simulink model "launch_controller_base"  (R2024b)
settings: Solver=VariableStepAuto  StartTime=0.0  StopTime=10.0  FixedStep=0.004  RelTol=1e-3
settings Model: Creator=lukec  LastModifiedBy=lukec
settings OptimizationCC: DefaultParameterBehavior=Inlined  EnhancedBackFolding=on  PassReuseOutputArgsAs=Individual arguments  ZeroExternalMemoryAtStartup=off  ZeroInternalMemoryAtStartup=off  OptimizeBlockOrder=speed  DifferentSizesBufferReuse=on  OptimizationCustomize=off  EfficientTunableParamExpr=on
settings DebuggingCC: ParameterTunabilityLossMsg=error
settings SFSimCC: MATLABDynamicMemAlloc=off
settings RTWCC: Description=Embedded Coder  SystemTargetFile=ert.tlc  GenCodeOnly=on  PackageGeneratedCodeAndArtifacts=on  TemplateMakefile=ert_default_tmf  Toolchain=CMake  TargetLang=C++
settings CodeAppCC: ForceParamTrailComments=on  IgnoreCustomStorageClasses=off  OperatorAnnotations=on  SimulinkDataObjDesc=on  SFDataObjDesc=on  InsertBlockDesc=on
settings ERTTargetCC: TargetLangStandard=C++11 (ISO)  GenerateSampleERTMain=on  CodeInterfacePackaging=C++ class  RootIOFormat=Structure reference  ERTCustomFileTemplate=example_file_process.tlc

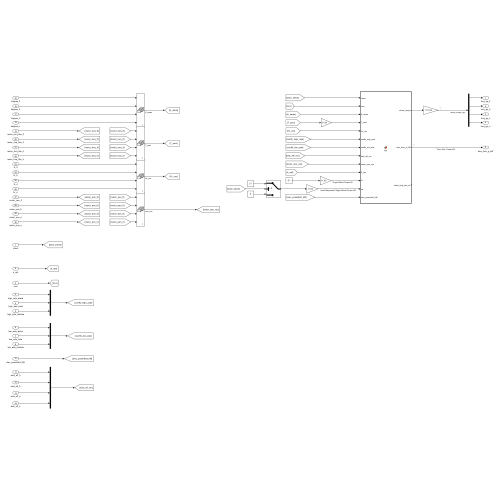
[thumbnail: Simulink's stored preview of the top-level diagram]
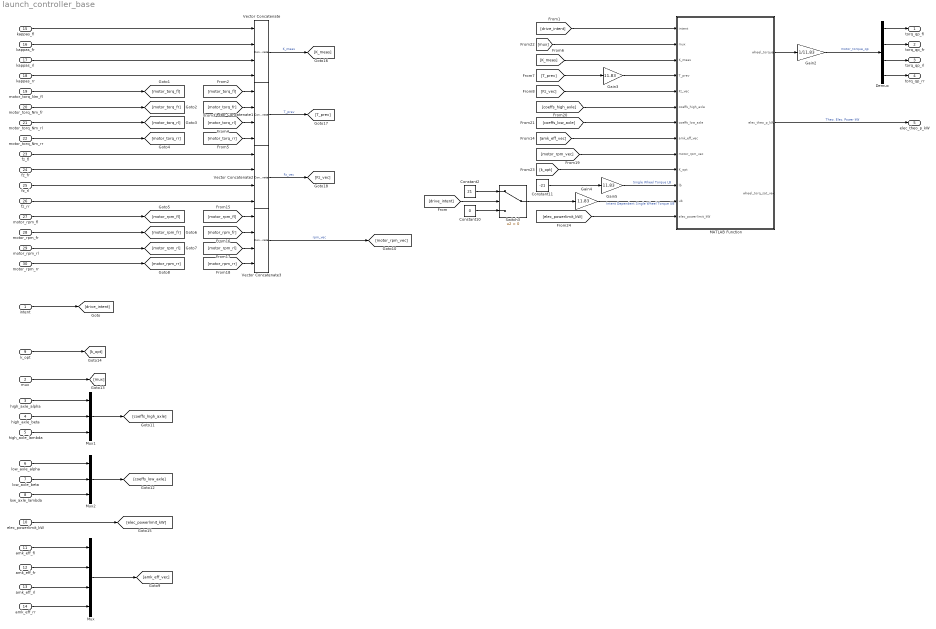
== system launch_controller_base ==
  intent : Inport
  mux : Inport  Port=2
  high_axle_alpha : Inport  Port=3
  high_axle_beta : Inport  Port=4
  high_axle_lambda : Inport  Port=5
  low_axle_alpha : Inport  Port=6
  low_axle_beta : Inport  Port=7
  low_axle_lambda : Inport  Port=8
  k_opt : Inport  Port=9
  elec_powerlimit_kW : Inport  Port=10
  amk_eff_fl : Inport  Port=11
  amk_eff_fr : Inport  Port=12
  amk_eff_rl : Inport  Port=13
  amk_eff_rr : Inport  Port=14
  kappas_fl : Inport  Port=15
  kappas_fr : Inport  Port=16
  kappas_rl : Inport  Port=17
  kappas_rr : Inport  Port=18
  motor_torq_Nm_fl : Inport  Port=19
  motor_torq_Nm_fr : Inport  Port=20
  motor_torq_Nm_rl : Inport  Port=21
  motor_torq_Nm_rr : Inport  Port=22
  fz_fl : Inport  Port=23
  fz_fr : Inport  Port=24
  fz_rl : Inport  Port=25
  fz_rr : Inport  Port=26
  motor_rpm_fl : Inport  Port=27
  motor_rpm_fr : Inport  Port=28
  motor_rpm_rl : Inport  Port=29
  motor_rpm_rr : Inport  Port=30
  Constant10 : Constant  Value=0
  Constant11 : Constant  Value=-21
  Constant2 : Constant  Value=21
  Demux : Demux
  Gain2 : Gain  Gain=1/11.83
  Gain3 : Gain  Gain=11.83
  Gain4 : Gain  Gain=11.83
  Gain5 : Gain  Gain=11.83
  MATLAB Function : MATLAB Function  TreatAsAtomicUnit=on
  Mux : Mux
  Mux1 : Mux  Inputs=3
  Mux2 : Mux  Inputs=3
  Switch3 : Switch  Criteria=u2 > Threshold  SaturateOnIntegerOverflow=off  InputSameDT=off
  Vector Concatenate{,1..3} (4 alike) : Concatenate  NumInputs=4  Mode=Multidimensional array
  torq_qp_fl : Outport
  torq_qp_fr : Outport  Port=2
  torq_qp_rl : Outport  Port=3
  torq_qp_rr : Outport  Port=4
  elec_theo_p_kW : Outport  Port=5
  wires:
  intent/1 -> [drive_intent]
  amk_eff_fl/1 -> Mux/1
  kappas_fr/1 -> Vector Concatenate/2
  motor_rpm_rl/1 -> [motor_rpm_rl]
  kappas_fl/1 -> Vector Concatenate/1
  motor_torq_Nm_fr/1 -> [motor_torq_fr]
  motor_torq_Nm_fl/1 -> [motor_torq_fl]
  motor_rpm_fr/1 -> [motor_rpm_fr]
  fz_rr/1 -> Vector Concatenate2/4
  fz_fr/1 -> Vector Concatenate2/2
  motor_torq_Nm_rl/1 -> [motor_torq_rl]
  amk_eff_rr/1 -> Mux/4
  amk_eff_fr/1 -> Mux/2
  [Fz_vec] -> MATLAB Function/5(Fz_vec)
  [drive_intent] -> Switch3/2
  low_axle_alpha/1 -> Mux2/1
  fz_rl/1 -> Vector Concatenate2/3
  [motor_torq_rl] -> Vector Concatenate1/3
  Gain2/1 -> Demux/1  "motor_torque_qp"
  motor_rpm_fl/1 -> [motor_rpm_fl]
  [k_opt] -> MATLAB Function/10(K_opt)
  [K_meas] -> MATLAB Function/3(K_meas)
  [motor_rpm_fr] -> Vector Concatenate3/2
  Gain3/1 -> MATLAB Function/4(T_prev)
  Mux/1 -> [amk_eff_vec]
  motor_rpm_rr/1 -> [motor_rpm_rr]
  low_axle_beta/1 -> Mux2/2
  [motor_torq_rr] -> Vector Concatenate1/4
  Demux/2 -> torq_qp_fr/1
  Vector Concatenate3/1 -> [motor_rpm_vec]  "rpm_vec"
  mux/1 -> [mux]
  high_axle_lambda/1 -> Mux1/3
  [motor_rpm_rr] -> Vector Concatenate3/4
  [motor_rpm_rl] -> Vector Concatenate3/3
  Gain4/1 -> MATLAB Function/12(ub)  "Intent Dependent Single Wheel Torque UB"
  Mux2/1 -> [coeffs_low_axle]
  Vector Concatenate/1 -> [K_meas]  "K_meas"
  MATLAB Function/2(elec_theo_p_kW) -> elec_theo_p_kW/1  "Theo. Elec. Power kW"
  [motor_torq_fr] -> Vector Concatenate1/2
  amk_eff_rl/1 -> Mux/3
  high_axle_alpha/1 -> Mux1/1
  [motor_rpm_fl] -> Vector Concatenate3/1
  elec_powerlimit_kW/1 -> [elec_powerlimit_kW]
  kappas_rr/1 -> Vector Concatenate/4
  k_opt/1 -> [k_opt]
  MATLAB Function/1(wheel_torque) -> Gain2/1
  high_axle_beta/1 -> Mux1/2
  [motor_torq_fl] -> Vector Concatenate1/1
  [motor_rpm_vec] -> MATLAB Function/9(motor_rpm_vec)
  Demux/3 -> torq_qp_rl/1
  Demux/1 -> torq_qp_fl/1
  motor_torq_Nm_rr/1 -> [motor_torq_rr]
  Mux1/1 -> [coeffs_high_axle]
  low_axle_lambda/1 -> Mux2/3
  Gain5/1 -> MATLAB Function/11(lb)  "Single Wheel Torque LB"
  [coeffs_high_axle] -> MATLAB Function/6(coeffs_high_axle)
  Constant11/1 -> Gain5/1
  [coeffs_low_axle] -> MATLAB Function/7(coeffs_low_axle)
  Switch3/1 -> Gain4/1
  Constant2/1 -> Switch3/1
  [amk_eff_vec] -> MATLAB Function/8(amk_eff_vec)
  fz_fl/1 -> Vector Concatenate2/1
  [elec_powerlimit_kW] -> MATLAB Function/13(elec_powerlimit_kW)
  [mux] -> MATLAB Function/2(mux)
  Vector Concatenate2/1 -> [Fz_vec]  "Fz_vec"
  Constant10/1 -> Switch3/3
  [drive_intent] -> MATLAB Function/1(intent)
  Vector Concatenate1/1 -> [T_prev]  "T_prev"
  kappas_rl/1 -> Vector Concatenate/3
  [T_prev] -> Gain3/1
  Demux/4 -> torq_qp_rr/1

== matlab function launch_controller_base/MATLAB Function ==
  data: intent input; mux input; K_meas input; wheel_torque output; T_prev input; Fz_vec input; coeffs_high_axle input; coeffs_low_axle input; amk_eff_vec input; motor_rpm_vec input; K_opt input; lb input; ub input; elec_theo_p_kW output; wheel_torq_sat_vec output; elec_powerlimit_kW input
function [wheel_torque, elec_theo_p_kW, wheel_torq_sat_vec] = fcn(intent, mux, K_meas, T_prev, Fz_vec, coeffs_high_axle, coeffs_low_axle, amk_eff_vec, motor_rpm_vec, K_opt, lb, ub, elec_powerlimit_kW)

    rpm2rad_s = 0.10472;

    lb = lb .* ones(4, 1);
    ub = ub .* ones(4, 1);

    r = 0.2;

    Fz_testpoints = [-100	-150	-200	-250	-300	-350	-400	-450	-500	-550	-600	-650	-700	-750	-800	-850	-900	-950	-1000	-1050	-1100	-1150	-1200	-1250	-1300	-1350	-1400	-1450	-1500	-1550	-1600	-1650	-1700	-1750	-1800	-1850	-1900	-1950	-2000] .* -1;
    CK_testpoints = [4993.96037580768	7230.15025002608	9312.63116671493	11255.0952723015	13070.0418608112	14768.7810353328	16361.4690854774	17857.1668314117	19263.9134694458	20588.8097872709	21838.1058844771	23017.2896709141	24131.1733923846	25183.9762444061	26179.4017891894	27120.7094051015	28010.7793914951	28852.1716449660	29647.1780346286	30397.8687505021	31106.1329947657	31773.7144422382	32402.2419235013	32993.2557891554	33548.2304026337	34068.5931861850	34555.7406132517	35011.0515026319	35435.8979267288	35831.6539982093	36199.7027460456	36541.4412318642	36858.2839884342	37151.6647804853	37423.0365888119	37673.8695948128	37905.6467846387	38119.8565869283	38317.9816880605];
    % wheel_torq_peak_testpoints = [52.1587700209819	76.7092632028708	100.090133113434	122.214122971230	143.039214005665	162.586784646041	180.951241062026	198.296774668120	214.840198965019	230.822876654010	246.477862335398	261.999366051929	277.520397915825	293.101807557612	308.732994265824	324.342198329281	339.812915440526	355.002646432221	369.760699142925	383.942767833758	397.421175370726	410.090684387646	421.870494543937	432.703401387688	442.553153546469	451.400911516527	459.241487408791	466.079809572184	471.927855032480	476.802144075737	480.721794639243	483.707079932916	485.778408828830	486.979471027242	487.420944353032	487.108400550003	486.059251779054	484.248903710396	481.702387075522];

    CK_vec = zeros(4, 1);
    wheel_torq_peak_vec = CK_vec;

    for i = 1:4
        
        if Fz_vec(i) < min(Fz_testpoints)
            Fz_vec(i) = min(Fz_testpoints);
        elseif Fz_vec(i) > max(Fz_testpoints)
            Fz_vec(i) = max(Fz_testpoints);
        end

        CK_vec(i) = interp1(Fz_testpoints', CK_testpoints', Fz_vec(i));
        wheel_torq_peak_vec(i) = Fz_vec(i) * mux * 0.2;
    end

    peak_net_wheel_torq = sum(wheel_torq_peak_vec);
    net_fz = sum(Fz_vec);
    perc_fz = abs(Fz_vec ./ net_fz);
    wheel_torq_sat_vec = perc_fz .* peak_net_wheel_torq;

    if intent >= 0

        alpha_vec = [coeffs_low_axle(1), coeffs_low_axle(1), coeffs_high_axle(1), coeffs_high_axle(1)];
        beta_vec = [coeffs_low_axle(2), coeffs_low_axle(2), coeffs_high_axle(2), coeffs_high_axle(2)];
        lambda_vec = [coeffs_low_axle(3), coeffs_low_axle(3), coeffs_high_axle(3), coeffs_high_axle(3)];

        lb = lb .* 0;

    else
        
        alpha_vec = [coeffs_high_axle(1), coeffs_high_axle(1), coeffs_low_axle(1), coeffs_low_axle(1)];
        beta_vec = [coeffs_high_axle(2), coeffs_high_axle(2), coeffs_low_axle(2), coeffs_low_axle(2)];
        lambda_vec = [coeffs_high_axle(3), coeffs_high_axle(3), coeffs_low_axle(3), coeffs_low_axle(3)];

        alpha_vec = abs(alpha_vec) .* -1;
        K_opt = abs(K_opt) * -1;
        ub = ub .* 0;

    end

    ele = zeros(4, 1);
    f = zeros(4, 1);

    for i = 1:4
        alpha = alpha_vec(i);
        beta = beta_vec(i);
        lambda = lambda_vec(i);

        CK = CK_vec(i);

        ele(i) = (beta / ((r * CK)^2)) + lambda;

        T_i_prev = T_prev(i);
        K_i_meas = K_meas(i);

        term1 = -alpha * (1 / (r * CK));

        term2_1 = (2 * (K_i_meas - K_opt)) / (r * CK);
        term2_2 = (-2 * T_i_prev) / ((r * CK)^2);
        term2 = beta * (term2_1 + term2_2);

        term3 = -2 *lambda * T_i_prev;

        f(i) = term1 + term2 + term3;
    end

    H = diag(ele) .* 2;


    A = zeros(1, 4);

    for i = 1:4
        A(i) = (motor_rpm_vec(i) * rpm2rad_s / amk_eff_vec(i)) / 11.83;
    end

    A = [A; diag([1 1 1 1]); diag(A)];

    if intent < 0
        A = A .* -1;
    end

    b = [elec_powerlimit_kW * 1000;
         wheel_torq_sat_vec;
         [33000; 33000; 33000; 33000]];

    % x0 = [0; 0; 0; 0];
    opts = optimoptions("quadprog", Algorithm="active-set");

    if intent ~= 0
        wheel_torque = quadprog(H, f, A, b, [], [], lb, ub, T_prev, opts);
    else
        wheel_torque = [0;0;0;0];
    end

    elec_theo_p_kW = (A(1, :) * wheel_torque) / 1000;
